simulink model "GSTA_FHGO"  (R2020a)
settings: Solver=VariableStepAuto  StartTime=0.0  StopTime=10  FixedStep=10e-3  RelTol=1e-3
settings Model: Creator=LENOVO PC  LastModifiedBy=LENOVO PC

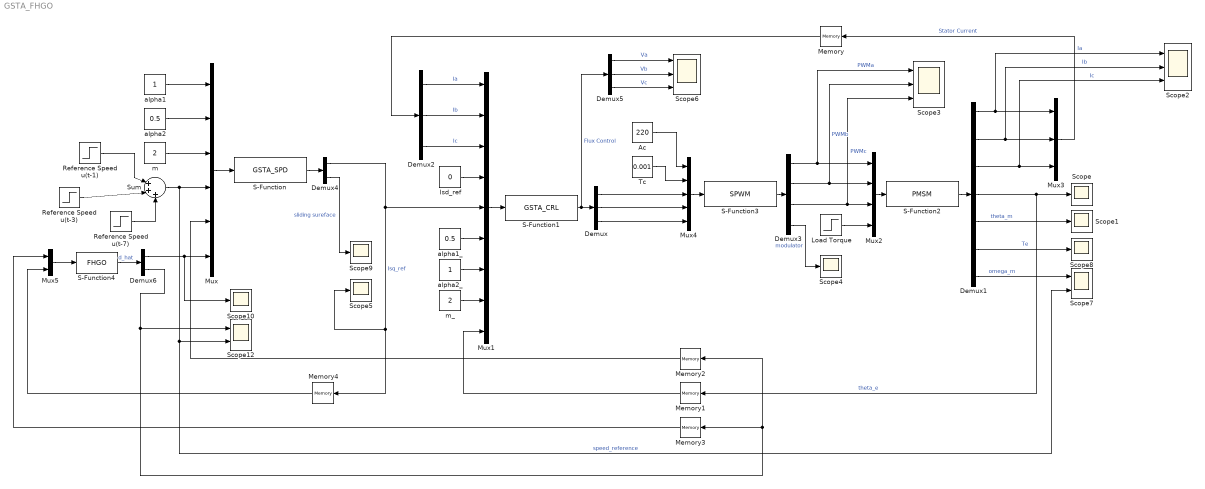
== system GSTA_FHGO ==
  Ac : Constant  Value=220
  Demux : Demux  Outputs=3
  Demux1 : Demux  Outputs=7
  Demux2 : Demux  Outputs=3
  Demux3 : Demux
  Demux4 : Demux  Outputs=2
  Demux5 : Demux  Outputs=3
  Demux6 : Demux  Outputs=2
  Isd_ref : Constant  Value=0
  Load Torque : Step  Time=0  After=5  SampleTime=0
  Memory{,1..4} (5 alike) : Memory
  Mux : Mux  Inputs=6
  Mux1 : Mux  Inputs=9
  Mux2 : Mux
  Mux3 : Mux  Inputs=3
  Mux4 : Mux  Inputs=5
  Mux5 : Mux  Inputs=2
  Reference Speed u(t-1) : Step  After=20  SampleTime=0
  Reference Speed u(t-3) : Step  Time=4  After=10  SampleTime=0
  Reference Speed u(t-7) : Step  Time=7  After=10  SampleTime=0
  S-Function : S-Function  FunctionName=GSTA_SPD  SFunctionDeploymentMode=off  EnableBusSupport=off
  S-Function1 : S-Function  FunctionName=GSTA_CRL  SFunctionDeploymentMode=off  EnableBusSupport=off
  S-Function2 : S-Function  FunctionName=PMSM  SFunctionDeploymentMode=off  EnableBusSupport=off
  S-Function3 : S-Function  FunctionName=SPWM  SFunctionDeploymentMode=off  EnableBusSupport=off
  S-Function4 : S-Function  FunctionName=FHGO  SFunctionDeploymentMode=off  EnableBusSupport=off
  Scope{,1,4..5,8..10} (7 alike) : Scope
  Scope12 : Scope  NumInputPorts=2
  Scope2 : Scope  NumInputPorts=3
  Scope3 : Scope  NumInputPorts=3
  Scope6 : Scope  NumInputPorts=3
  Scope7 : Scope  NumInputPorts=2
  Sum : Sum  Inputs=|+++
  Tc : Constant  Value=0.001
  alpha1 : Constant
  alpha1_ : Constant  Value=0.5
  alpha2 : Constant  Value=0.5
  alpha2_ : Constant
  m : Constant  Value=2
  m_ : Constant  Value=2
  wires:
  Mux/1 -> S-Function/1
  Mux4/1 -> S-Function3/1
  alpha2/1 -> Mux/2
  Memory2/1 -> Mux/5
  Memory/1 -> Demux2/1
  Mux2/1 -> S-Function2/1
  Demux1/3 -> Mux3/3, Scope2/3  "Ic"
  Ac/1 -> Mux4/1
  Demux2/1 -> Mux1/1  "Ia"
  Demux2/2 -> Mux1/2  "Ib"
  Mux3/1 -> Memory/1  "Stator Current"
  Demux1/2 -> Scope2/2, Mux3/2  "Ib"
  S-Function2/1 -> Demux1/1
  alpha1/1 -> Mux/1
  Demux1/1 -> Scope2/1, Mux3/1  "Ia"
  Load Torque/1 -> Mux2/4
  Demux2/3 -> Mux1/3  "Ic"
  S-Function1/1 -> Demux/1, Demux5/1  "Flux Control"
  S-Function3/1 -> Demux3/1
  Mux1/1 -> S-Function1/1
  Demux1/4 -> Memory1/1, Scope/1  "theta_e"
  Demux1/5 -> Scope1/1  "theta_m"
  Demux1/6 -> Scope8/1  "Te"
  Demux1/7 -> Scope7/1  "omega_m"
  Demux/3 -> Mux4/5
  Demux/2 -> Mux4/4
  Demux/1 -> Mux4/3
  Tc/1 -> Mux4/2
  Demux3/1 -> Mux2/1, Scope3/1  "PWMa"
  Demux3/2 -> Mux2/2, Scope3/2  "PWMb"
  Demux3/3 -> Scope3/3, Mux2/3  "PWMc"
  Demux3/4 -> Scope4/1  "modulator"
  Isd_ref/1 -> Mux1/4
  Memory1/1 -> Mux1/9
  Demux5/1 -> Scope6/1  "Va"
  Demux5/2 -> Scope6/2  "Vb"
  Demux5/3 -> Scope6/3  "Vc"
  m/1 -> Mux/3
  S-Function/1 -> Demux4/1
  Demux4/1 -> Scope5/1, Memory4/1, Mux1/5  "Isq_ref"
  Demux4/2 -> Scope9/1  "sliding sureface"
  Mux5/1 -> S-Function4/1
  Memory4/1 -> Mux5/2
  Memory3/1 -> Mux5/1
  m_/1 -> Mux1/8
  alpha2_/1 -> Mux1/7
  alpha1_/1 -> Mux1/6
  Reference Speed u(t-3)/1 -> Sum/2
  Reference Speed u(t-1)/1 -> Sum/1
  Sum/1 -> Mux/4, Scope12/2, Scope7/2  "speed_reference"
  Reference Speed u(t-7)/1 -> Sum/3
  S-Function4/1 -> Demux6/1  "d_hat"
  Demux6/1 -> Scope10/1, Mux/6
  Demux6/2 -> Scope12/1, Memory2/1, Memory3/1
